simulink model "performance_task"  (R2016a)
settings: Solver=VariableStepAuto  StartTime=0.0  StopTime=2  RelTol=1e-3
libraries: dsparch4 x1
settings Model: Creator=SHADRIL HASSAN  LastModifiedBy=SHADRIL HASSAN

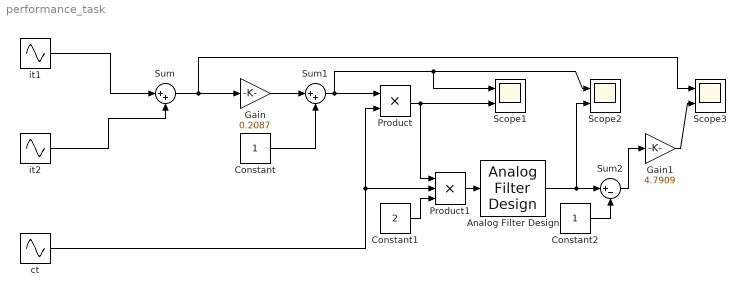
== system performance_task ==
  Analog Filter Design : dsparch4/Analog Filter Design  method=Butterworth  filttype=Lowpass  N=10  Wlo=2*pi*9  Whi=80  Rp=2  Rs=40
  Constant : Constant
  Constant1 : Constant  Value=2
  Constant2 : Constant
  Gain : Gain  Gain=0.2087
  Gain1 : Gain  Gain=4.7909
  Product : Product
  Product1 : Product  Inputs=3
  Scope1 : Scope  NumInputPorts=2
  Scope2 : Scope  NumInputPorts=2
  Scope3 : Scope  NumInputPorts=2
  Sum : Sum  Inputs=|++
  Sum1 : Sum  Inputs=|++
  Sum2 : Sum  Inputs=|+-
  ct : Sin  Frequency=2*pi*50  Phase=pi/2  SampleTime=1/10000
  it1 : Sin  Amplitude=2  Frequency=2*pi*4  SampleTime=1/10000
  it2 : Sin  Amplitude=3  Frequency=2*pi*6  Phase=pi/2  SampleTime=1/10000
  wires:
  it1/1 -> Sum/1
  it2/1 -> Sum/2
  Gain/1 -> Sum1/1
  Constant/1 -> Sum1/2
  Sum/1 -> Scope3/1, Gain/1
  Sum1/1 -> Scope1/1, Scope2/1, Product/1
  ct/1 -> Product1/2, Product/2
  Product/1 -> Scope1/2, Product1/1
  Constant1/1 -> Product1/3
  Product1/1 -> Analog Filter Design/1
  Analog Filter Design/1 -> Sum2/1, Scope2/2
  Constant2/1 -> Sum2/2
  Sum2/1 -> Gain1/1
  Gain1/1 -> Scope3/2
